simulink model "mod_5_counter"  (R2020b)
settings: Solver=VariableStepAuto  StartTime=0.0  StopTime=50  RelTol=1e-3
settings Model: Creator=153  LastModifiedBy=153

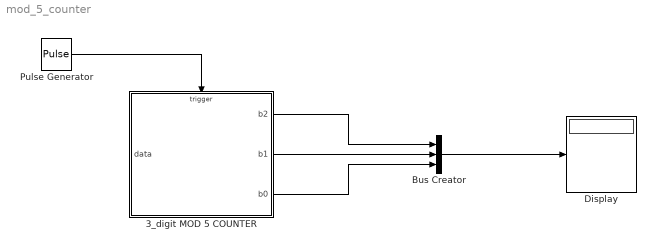
== system mod_5_counter ==
  3_digit MOD 5 COUNTER : Stateflow chart  TreatAsAtomicUnit=on
  Bus Creator : BusCreator  Inputs=3
  Display : Display
  Pulse Generator : DiscretePulseGenerator  PulseType=Time based  Period=1  PulseWidth=5
  wires:
  3_digit MOD 5 COUNTER/1(b2) -> Bus Creator/1
  3_digit MOD 5 COUNTER/2(b1) -> Bus Creator/2
  3_digit MOD 5 COUNTER/3(b0) -> Bus Creator/3
  Bus Creator/1 -> Display/1
  Pulse Generator/1 -> 3_digit MOD 5 COUNTER/Trigger

== stateflow chart mod_5_counter/3_digit MOD 5 COUNTER ==
  settings: executeAtInitialization=1
  state digit0 [parallel]
    settings: executionOrder=3
    state bit1
      en: b0=1;
    state bit0
      en: b0=0;
    bit0 -> bit1 : bit0_event
    bit1 -> bit0 : bit0_event
    (default) -> bit0
  state digit1 [parallel]
    settings: executionOrder=2
    state bitt
      en: b1=1;
    state bit
      en: b1=0;
    bit -> bitt : bit1_event[in(check.inflow)]
    bitt -> bit : bit1_event/{digit0.bit0_event;}
    (default) -> bit
  state digit2 [parallel]
    settings: executionOrder=1
    state bit3
      en: b2=1;
    state bit2
      en: b2=0;
    bit2 -> bit3 : r_event[in(check.inflow)]
    bit3 -> bit2 : r_event/{digit1.bit1_event;}
    (default) -> bit2
  state check [parallel]
    settings: executionOrder=4
    state overflow
    state inflow
    (default) -> inflow
    overflow -> inflow : [ in(digit1.bitt)]
    inflow -> overflow : [in(digit0.bit1) && in(digit1.bit)]
  data: b2 output size=1; b1 output size=1; b0 output size=1; data input
  events: bit0_event local FUNCTION_CALL_EVENT; bit1_event local FUNCTION_CALL_EVENT; r_event input RISING_EDGE_EVENT
